simulink model "pendulo_inv_sim"  (R2024b)
settings: Solver=VariableStepAuto  StartTime=0.0  StopTime=15  MaxStep=0.01  RelTol=1e-3
InitFcn:
  | Ip = 0.0079;
  | Mc = 0.7031;
  | lp = 0.3302;
  | Mp = 0.23;
  | Fc = 0;
  | Beq = 4.3;
  | g = 9.81;
  | Bp = 0.0024;

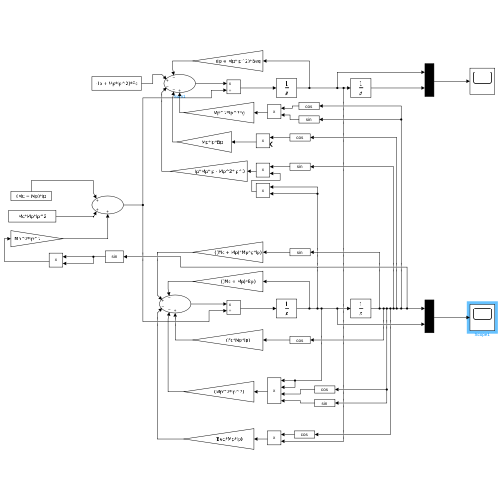
[thumbnail: Simulink's stored preview of the top-level diagram]
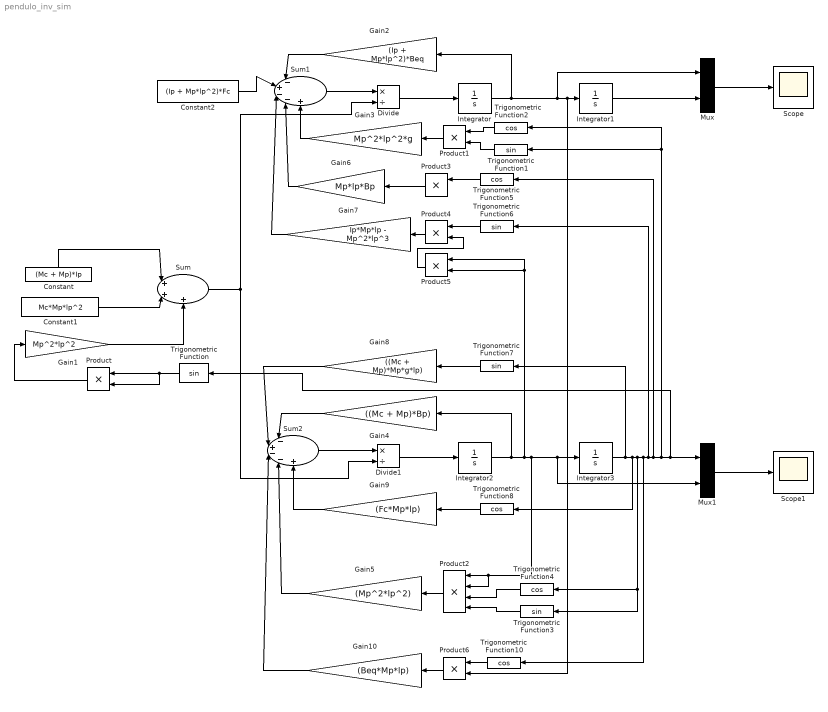
== system pendulo_inv_sim ==
  Constant : Constant  Value=(Mc + Mp)*Ip
  Constant1 : Constant  Value=Mc*Mp*lp^2
  Constant2 : Constant  Value=(Ip + Mp*lp^2)*Fc
  Divide : Product  Inputs=*/
  Divide1 : Product  Inputs=*/
  Gain1 : Gain  Gain=Mp^2*lp^2
  Gain10 : Gain  Gain=(Beq*Mp*lp)
  Gain2 : Gain  Gain=(Ip + Mp*lp^2)*Beq
  Gain3 : Gain  Gain=Mp^2*lp^2*g
  Gain4 : Gain  Gain=((Mc + Mp)*Bp)
  Gain5 : Gain  Gain=(Mp^2*lp^2)
  Gain6 : Gain  Gain=Mp*lp*Bp
  Gain7 : Gain  Gain=Ip*Mp*lp - Mp^2*lp^3
  Gain8 : Gain  Gain=((Mc + Mp)*Mp*g*lp)
  Gain9 : Gain  Gain=(Fc*Mp*lp)
  Integrator : Integrator
  Integrator1 : Integrator
  Integrator2 : Integrator
  Integrator3 : Integrator  InitialCondition=0.017453
  Mux : Mux  Inputs=2
  Mux1 : Mux  Inputs=2
  Product{,1,3..6} (6 alike) : Product
  Product2 : Product  Inputs=4
  Scope : Scope
  Scope1 : Scope
  Sum : Sum  Inputs=|+++
  Sum1 : Sum  Inputs=|-+--+
  Sum2 : Sum  Inputs=|-+--+
  Trigonometric Function{,1,3,6..7} (5 alike) : Trigonometry
  Trigonometric Function{2,4..5,8,10} (5 alike) : Trigonometry  Operator=cos
  wires:
  Trigonometric Function/1 -> Product/2, Product/1
  Product/1 -> Gain1/1
  Constant/1 -> Sum/1
  Constant1/1 -> Sum/2
  Gain1/1 -> Sum/3
  Sum1/1 -> Divide/1
  Divide/1 -> Integrator/1
  Integrator/1 -> Gain2/1, Mux/1, Product6/2, Integrator1/1
  Gain2/1 -> Sum1/1
  Constant2/1 -> Sum1/2
  Product1/1 -> Gain3/1
  Trigonometric Function2/1 -> Product1/1
  Trigonometric Function1/1 -> Product1/2
  Integrator1/1 -> Mux/2
  Product2/1 -> Gain5/1
  Sum2/1 -> Divide1/1
  Integrator2/1 -> Gain4/1, Product5/1, Product5/2, Product2/2, Product2/1, Mux1/2, Integrator3/1
  Divide1/1 -> Integrator2/1
  Product3/1 -> Gain6/1
  Gain3/1 -> Sum1/5
  Gain6/1 -> Sum1/4
  Trigonometric Function5/1 -> Product3/1
  Gain7/1 -> Sum1/3
  Product4/1 -> Gain7/1
  Trigonometric Function6/1 -> Product4/1
  Product5/1 -> Product4/2
  Integrator3/1 -> Trigonometric Function7/1, Trigonometric Function8/1, Trigonometric Function3/1, Trigonometric Function4/1, Trigonometric Function10/1, Trigonometric Function6/1, Trigonometric Function5/1, Trigonometric Function2/1, Trigonometric Function1/1, Trigonometric Function/1, Mux1/1
  Trigonometric Function7/1 -> Gain8/1
  Gain8/1 -> Sum2/2
  Gain4/1 -> Sum2/1
  Trigonometric Function8/1 -> Gain9/1
  Gain9/1 -> Sum2/5
  Trigonometric Function10/1 -> Product6/1
  Product6/1 -> Gain10/1
  Gain5/1 -> Sum2/4
  Gain10/1 -> Sum2/3
  Trigonometric Function3/1 -> Product2/4
  Trigonometric Function4/1 -> Product2/3
  Sum/1 -> Divide1/2, Divide/2
  Mux/1 -> Scope/1
  Mux1/1 -> Scope1/1
